simulink model "sim_2dof"  (R2024b)
settings: Solver=ode4  StartTime=t_0  StopTime=t_f  FixedStep=dt  RelTol=1e-8
undefined symbols (not defined in the file or in its folder): DRAG_DATA, GRAVITY, GROUND_LEVEL, MASS_DRY, position_init, REF_AREA, velocity_init
libraries: aerolibatmos2 x1
settings Model: Creator=yevge  LastModifiedBy=yevge
settings DebuggingCC: AlgebraicLoopMsg=error  CheckMatrixSingularityMsg=error

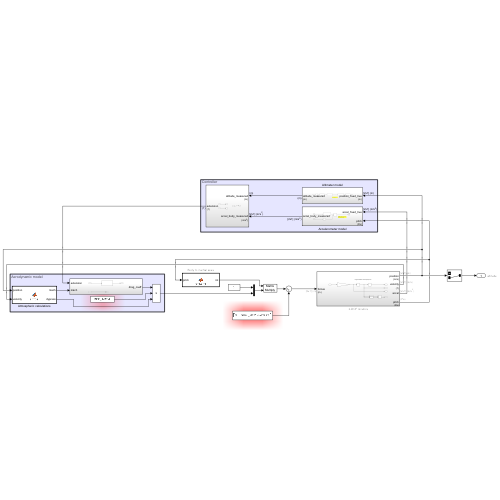
[thumbnail: Simulink's stored preview of the top-level diagram]
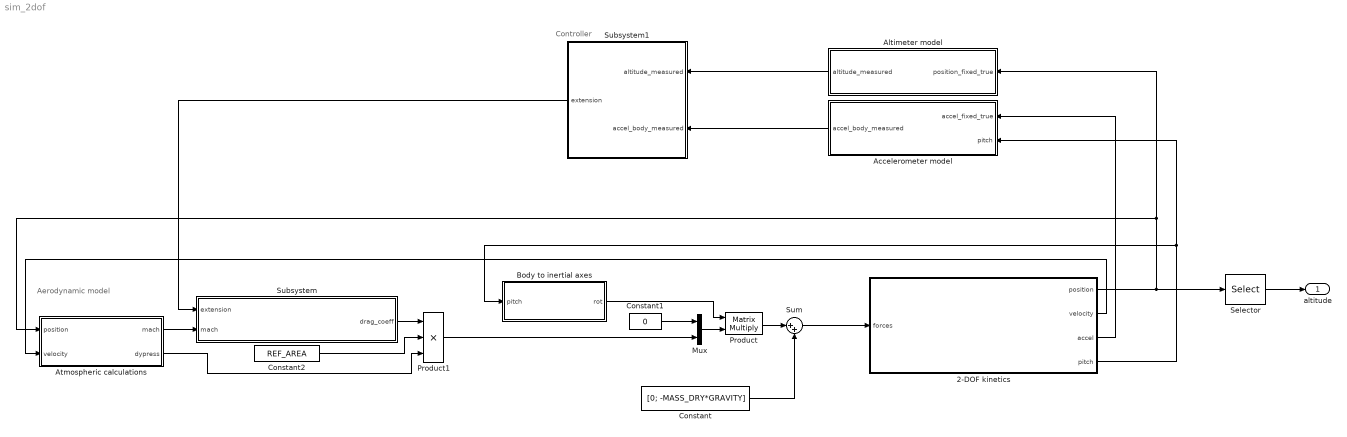
== system sim_2dof ==
  note: Aerodynamic model
  note: Controller
  2-DOF kinetics : Subsystem
  Accelerometer model : Subsystem
  Altimeter model : Subsystem
  Atmospheric calculations : MATLAB Function  TreatAsAtomicUnit=on
  Body to inertial axes : MATLAB Function  TreatAsAtomicUnit=on
  Constant : Constant  Value=[0; -MASS_DRY*GRAVITY]
  Constant1 : Constant  Value=0
  Constant2 : Constant  Value=REF_AREA
  Mux : Mux  Inputs=2
  Product : Product  Multiplication=Matrix(*)
  Product1 : Product  Inputs=3
  Selector : Selector  InputPortWidth=2  IndexOptions=Index vector (dialog)  Indices=2  OutputSizes=1
  Subsystem : Subsystem
  Subsystem1 : Subsystem
  Sum : Sum  Inputs=|++
  altitude : Outport
  wires:
  2-DOF kinetics/2(velocity) -> Atmospheric calculations/2(velocity)
  2-DOF kinetics/1(position) -> Selector/1, Atmospheric calculations/1(position), Altimeter model/1(position_fixed_true)
  2-DOF kinetics/4(pitch) -> Accelerometer model/2(pitch), Body to inertial axes/1(pitch)
  Sum/1 -> 2-DOF kinetics/1(forces)
  Product/1 -> Sum/1
  Body to inertial axes/1(rot) -> Product/1
  Mux/1 -> Product/2
  Constant1/1 -> Mux/1
  Product1/1 -> Mux/2
  Atmospheric calculations/2(dypress) -> Product1/3
  Constant2/1 -> Product1/2
  Constant/1 -> Sum/2
  Subsystem/1(drag_coeff) -> Product1/1
  Atmospheric calculations/1(mach) -> Subsystem/2(mach)
  2-DOF kinetics/3(accel) -> Accelerometer model/1(accel_fixed_true)
  Subsystem1/1(extension) -> Subsystem/1(extension)
  Altimeter model/1(altitude_measured) -> Subsystem1/1(altitude_measured)
  Accelerometer model/1(accel_body_measured) -> Subsystem1/2(accel_body_measured)
  Selector/1 -> altitude/1

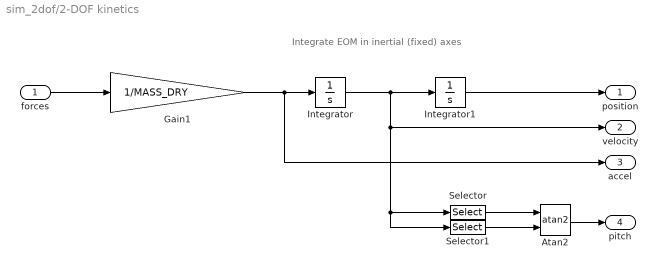
== system sim_2dof/2-DOF kinetics ==
  note: Integrate EOM in inertial (fixed) axes
  forces : Inport  Unit=N  PortDimensions=[2 1]
  Atan2 : Trigonometry  Operator=atan2
  Gain1 : Gain  Gain=1/MASS_DRY
  Integrator : Integrator  InitialCondition=velocity_init  ContinuousStateAttributes='velocity'
  Integrator1 : Integrator  InitialCondition=position_init  ContinuousStateAttributes='position'
  Selector : Selector  InputPortWidth=2  IndexOptions=Index vector (dialog)  Indices=2  OutputSizes=1
  Selector1 : Selector  InputPortWidth=2  IndexOptions=Index vector (dialog)  Indices=1  OutputSizes=1
  position : Outport  Unit=m  PortDimensions=[2 1]
  velocity : Outport  Port=2  Unit=m/s  PortDimensions=[2 1]
  accel : Outport  Port=3  Unit=m/s^2  PortDimensions=[2 1]
  pitch : Outport  Port=4  Unit=rad  PortDimensions=1
  wires:
  Integrator/1 -> Selector1/1, Selector/1, velocity/1, Integrator1/1
  Gain1/1 -> accel/1, Integrator/1
  forces/1 -> Gain1/1
  Integrator1/1 -> position/1
  Selector/1 -> Atan2/1
  Selector1/1 -> Atan2/2
  Atan2/1 -> pitch/1

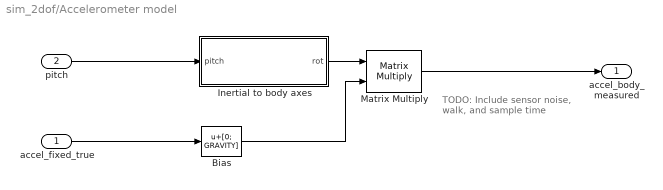
== system sim_2dof/Accelerometer model ==
  note: TODO: Include sensor noise, walk, and sample time
  accel_fixed_true : Inport  Unit=m/s^2  PortDimensions=[2 1]
  pitch : Inport  Port=2  Unit=rad  PortDimensions=1
  Bias : Bias  Bias=[0; GRAVITY]  SaturateOnIntegerOverflow=off
  Inertial to body axes : MATLAB Function  TreatAsAtomicUnit=on
  Matrix Multiply : Product  Multiplication=Matrix(*)
  accel_body_measured : Outport  Unit=m/s^2  PortDimensions=[2 1]
  wires:
  pitch/1 -> Inertial to body axes/1(pitch)
  Inertial to body axes/1(rot) -> Matrix Multiply/1
  accel_fixed_true/1 -> Bias/1
  Matrix Multiply/1 -> accel_body_measured/1
  Bias/1 -> Matrix Multiply/2

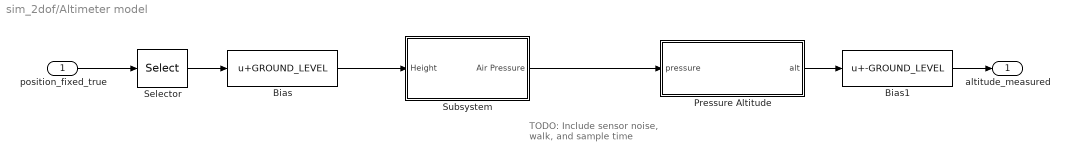
== system sim_2dof/Altimeter model ==
  note: TODO: Include sensor noise, walk, and sample time
  position_fixed_true : Inport  Unit=m  PortDimensions=[2 1]
  Bias : Bias  Bias=GROUND_LEVEL  SaturateOnIntegerOverflow=off
  Bias1 : Bias  Bias=-GROUND_LEVEL  SaturateOnIntegerOverflow=off
  Pressure Altitude : MATLAB Function  TreatAsAtomicUnit=on
  Selector : Selector  InputPortWidth=2  IndexOptions=Index vector (dialog)  Indices=2  OutputSizes=1
  Subsystem : Subsystem
      mask Display:
      | block_icon("ISA Atmosphere Model")
      | 
      | %text(0.5 , 0.3, "ISA Pressure", ...
      | %    HorizontalAlignment="center", VerticalAlignment="middle")
      | disp("\n\n\nISA Pressure");
  altitude_measured : Outport  Unit=m  PortDimensions=1
  wires:
  position_fixed_true/1 -> Selector/1
  Selector/1 -> Bias/1
  Pressure Altitude/1(alt) -> Bias1/1
  Bias1/1 -> altitude_measured/1
  Bias/1 -> Subsystem/1(Height)
  Subsystem/1(Air Pressure) -> Pressure Altitude/1(pressure)

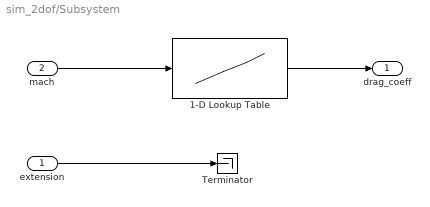
== system sim_2dof/Subsystem ==
  extension : Inport
  mach : Inport  Port=2
  1-D Lookup Table : Lookup_n-D  NumberOfTableDimensions=1  BreakpointsForDimension1=DRAG_DATA.MACH  Table=DRAG_DATA.DRAG  ExtrapMethod=Clip  UseLastTableValue=on  InternalRulePriority=Speed  RndMeth=Simplest
  Terminator : Terminator
  drag_coeff : Outport
  wires:
  extension/1 -> Terminator/1
  mach/1 -> 1-D Lookup Table/1
  1-D Lookup Table/1 -> drag_coeff/1

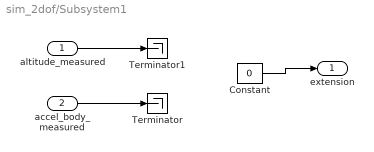
== system sim_2dof/Subsystem1 ==
  altitude_measured : Inport  Unit=m  PortDimensions=1
  accel_body_measured : Inport  Port=2  Unit=m/s^2  PortDimensions=[2 1]
  Constant : Constant  Value=0
  Terminator : Terminator
  Terminator1 : Terminator
  extension : Outport  OutMin=0  OutMax=1  Unit=1  PortDimensions=1
  wires:
  accel_body_measured/1 -> Terminator/1
  altitude_measured/1 -> Terminator1/1
  Constant/1 -> extension/1

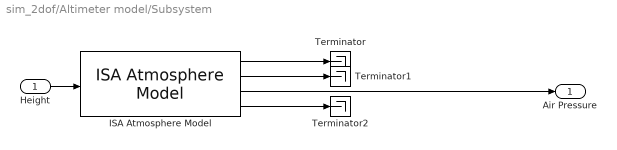
== system sim_2dof/Altimeter model/Subsystem ==
  Height : Inport
  ISA Atmosphere Model : aerolibatmos2/ISA Atmosphere Model  useExtended=off  action=Warning  custom=off  viscosityOut=off  g=9.80665  gamma=1.4  R=287.0531  L=0.0065  h_trop=11000  h_strat=20000  rho0=1.225  P0=101325  T0=288.15  h0=0  S=110.4  Tref=273.15  muref=1.716e-5
  Terminator : Terminator
  Terminator1 : Terminator
  Terminator2 : Terminator
  Air Pressure : Outport
  wires:
  ISA Atmosphere Model/1 -> Terminator/1
  ISA Atmosphere Model/3 -> Air Pressure/1
  ISA Atmosphere Model/2 -> Terminator1/1
  ISA Atmosphere Model/4 -> Terminator2/1
  Height/1 -> ISA Atmosphere Model/1

== matlab function sim_2dof/Body to inertial axes ==
  data: pitch input size=1; rot output size=[2 2]
function rot = pitch2rot(pitch)
    ct = cos(pitch);
    st = sin(pitch);
    rot = [ct st
        -st ct];
end

== matlab function sim_2dof/Atmospheric calculations ==
  data: position input size=[2 1]; mach output size=1; velocity input size=[2 1]; dypress output size=1; GROUND_LEVEL parameter size=1
function [mach, dypress] = atmos(position, velocity, ...
    GROUND_LEVEL)
    [~, a, ~, rho] = atmosisa(position(2) + GROUND_LEVEL);
    total_vel = vecnorm(velocity, 2, 1);
    mach = total_vel / a;
    dypress = 0.5 * rho * total_vel^2;
end

== matlab function sim_2dof/Accelerometer model/Inertial to body axes ==
  data: pitch input size=1; rot output size=[2 2]
function rot = pitch2rot(pitch)
    ct = cos(pitch);
    st = sin(pitch);
    rot = [ct st
        -st ct];
end

== matlab function sim_2dof/Altimeter model/Pressure Altitude ==
  data: pressure input; alt output
function alt = pressure_altitude(pressure)
    alt = (1 - (pressure ./ 101325).^(0.190284)) .* 145366.45 * 0.3048;
end
